simulink subsystem "thermal_stack_heat_emulation"  (R2023a)
settings: Solver=VariableStepAuto  StartTime=0.0  StopTime=10.0  RelTol=1e-3
values from neighbouring files (symbols this model uses):
  coolant_initial_temperature = 293.15    [thermal_model_parameters.m]    (also in thermal_plant_h2f175_parameters.m)
undefined symbols (not defined in the file or in its folder): stack
libraries: fl_lib x5, nesl_utility x2
settings Model: Creator=stefan.notter  LastModifiedBy=stefan.notter

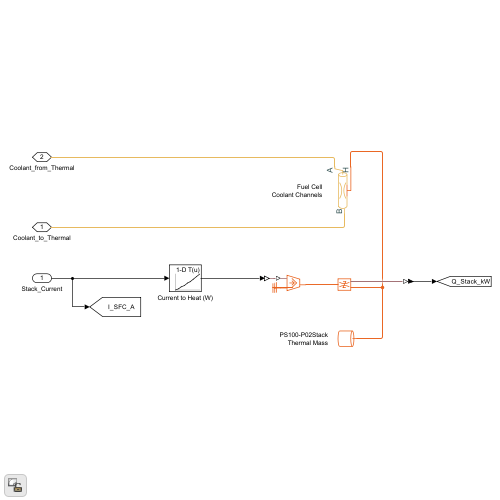
[thumbnail: Simulink's stored preview of the top-level diagram]
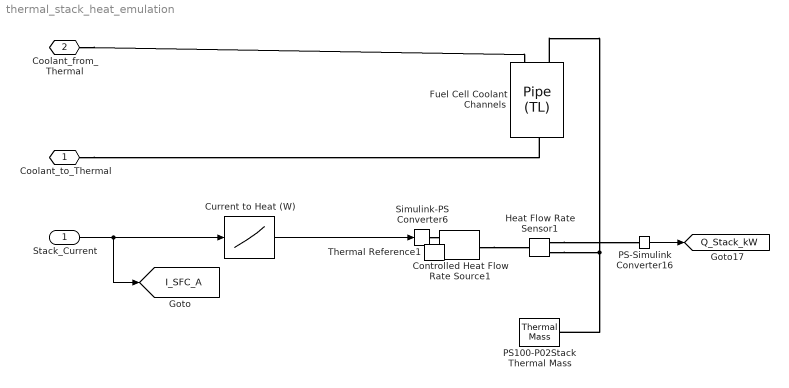
== system thermal_stack_heat_emulation ==
  Stack_Current : Inport
  Controlled Heat Flow Rate Source1 : fl_lib/Thermal/Thermal Sources/Controlled Heat Flow Rate Source
  Current to Heat (W) : Lookup_n-D  NumberOfTableDimensions=1  BreakpointsForDimension1=[0:50:400]  Table=[0, 9932, 21438, 33442,47123, 59491, 77033, 93585, 112042]  InternalRulePriority=Speed  RndMeth=Simplest
  Fuel Cell Coolant Channels : fl_lib/Thermal Liquid/Elements/Pipe (TL)  length=sqrt(stack.area) * stack.coolant_num_passes cm  area=stack.coolant_w_channels^2 * stack.coolant_num_layers cm^2  Dh=stack.coolant_w_channels cm  length_add=10 cm  roughness=15e-5 m  Re_lam=2000  Re_tur=4000  shape_factor=64  Nu_lam=3.66  dynamic_compressibility=simscape.enum.onoff.on  inertia=simscape.enum.onoff.off  p0=coolant_initial_pressure MPa  T0=coolant_initial_temperature K  mdot0=0 kg/s
  Heat Flow Rate Sensor1 : fl_lib/Thermal/Thermal Sensors/Heat Flow Rate Sensor
  PS-Simulink Converter16 : nesl_utility/PS-Simulink Converter  PhysicalDomain=network_engine_domain  SubClassName=ps_output  LeftPortType=input  RightPortType=output  PseudoPeriodic=off  Frequencies=[]  VectorFormat=1-D array  Unit=kW  AffineConversion=off
  PS100-P02Stack Thermal Mass : fl_lib/Thermal/Thermal Elements/Thermal Mass  mass_type=foundation.enum.constant_variable.constant  mass=stack.thermal_mass kg  sp_heat=stack.specific_heat J/kg/K  mass_min=1e-6 kg  num_ports=foundation.enum.numPorts2.one  m_specify=off  m_priority=High  m=1 kg  m_nominal_specify=off  m_nominal_unit=kg  m_nominal_value=1  T_specify=on  T_priority=High  T=coolant_initial_temperature K  T_nominal_specify=off  T_nominal_unit=K  T_nominal_value=1  Q_specify=off  Q_priority=None  Q=20e3 W  Q_nominal_specify=off  Q_nominal_unit=W  Q_nominal_value=1
  Simulink-PS Converter6 : nesl_utility/Simulink-PS Converter  PhysicalDomain=network_engine_domain  SubClassName=ps_input  LeftPortType=input  RightPortType=output  PseudoPeriodic=off  Frequencies=[]  NoiseDistribution=none  NoiseParameters=[]  Unit=J/s  AffineConversion=off  FilteringAndDerivatives=provide  SimscapeFilterOrder=1  InputFilterTimeConstant=0.001  UdotUserProvided=0
  Thermal Reference1 : fl_lib/Thermal/Thermal Elements/Thermal Reference
  Coolant_to_Thermal : PMIOPort  Side=Right
  Coolant_from_Thermal : PMIOPort  Port=2  Side=Right
  tag scope: I_SFC_A=global, Q_Stack_kW=global
  wires:
  PS-Simulink Converter16/1 -> [Q_Stack_kW]
  Stack_Current/1 -> [I_SFC_A], Current to Heat (W)/1
  Current to Heat (W)/1 -> Simulink-PS Converter6/1
  connections:
  Heat Flow Rate Sensor1/RConn2 -- Fuel Cell Coolant Channels/LConn2 -- PS100-P02Stack Thermal Mass/LConn1
  Thermal Reference1/LConn1 -- Controlled Heat Flow Rate Source1/RConn2
  Controlled Heat Flow Rate Source1/LConn1 -- Heat Flow Rate Sensor1/LConn1
  Heat Flow Rate Sensor1/RConn1 -- PS-Simulink Converter16/LConn1
  Simulink-PS Converter6/RConn1 -- Controlled Heat Flow Rate Source1/RConn1
  Coolant_from_Thermal/RConn1 -- Fuel Cell Coolant Channels/LConn1
  Coolant_to_Thermal/RConn1 -- Fuel Cell Coolant Channels/RConn1
